simulink model "StateMachine_MR"  (R2013a)
settings: Solver=FixedStepDiscrete  StartTime=0.0  StopTime=10.0  RelTol=1e-3
settings Model: Creator=shipmanr  LastModifiedBy=shipmanr

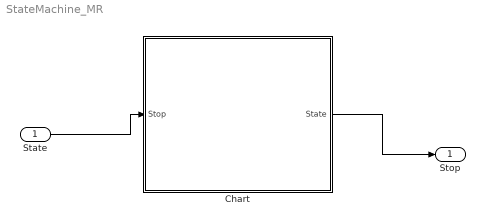
== system StateMachine_MR ==
  State : Inport
  Chart : Stateflow chart  TreatAsAtomicUnit=on
  Stop : Outport
  wires:
  State/1 -> Chart/1(Stop)
  Chart/1(State) -> Stop/1

== stateflow chart StateMachine_MR/Chart ==
  state Wait
    entry:
    State=RobotState.Wait;
  state Stop
    entry:
    State=RobotState.Stop;
  (default) -> Wait
  Wait -> Stop : [Stop]
  data: Stop input; State output double
